simulink subsystem "WB"  (R2024b)
settings: Solver=VariableStepAuto  StartTime=0.0  StopTime=10.0  RelTol=1e-3
libraries: hdlsllib x1
settings Model: Creator=stefano  LastModifiedBy=stefano

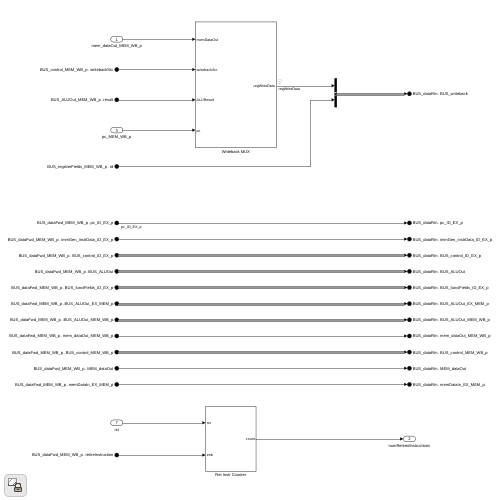
[thumbnail: Simulink's stored preview of the top-level diagram]
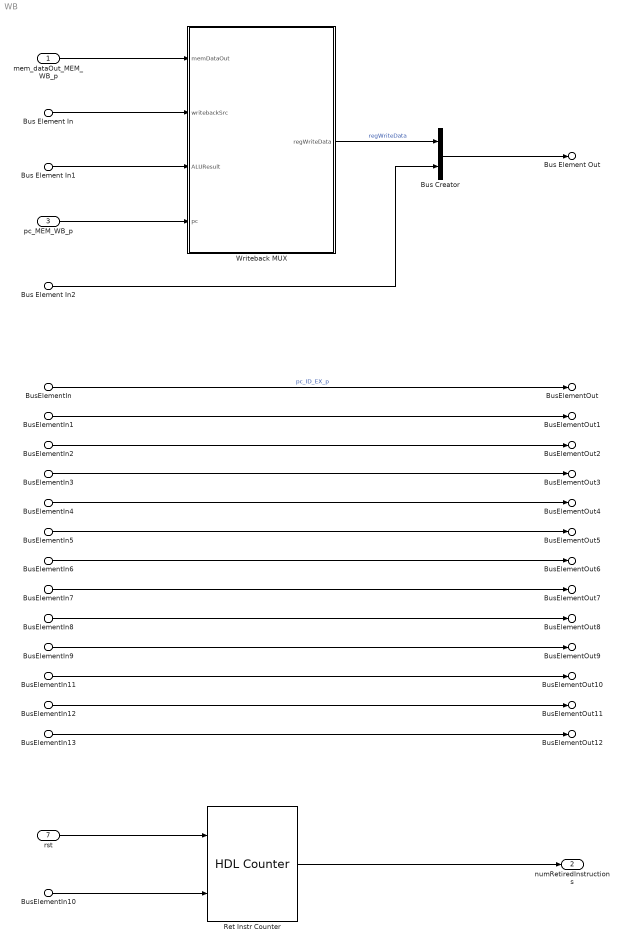
== system WB ==
  mem_dataOut_MEM_WB_p : Inport
  Bus Element In1 : Inport  Port=2  PortName=BUS_ALUOut_MEM_WB_p  Element=result
  pc_MEM_WB_p : Inport  Port=3
  Bus Element In : Inport  Port=4  PortName=BUS_control_MEM_WB_p  Element=writebackSrc
  Bus Element In2 : Inport  Port=5  PortName=BUS_registerFields_MEM_WB_p  Element=rd
  BusElementIn : Inport  Port=6  PortName=BUS_dataFwd_MEM_WB_p  Element=pc_ID_EX_p
  BusElementIn1 : Inport  Port=6  PortName=BUS_dataFwd_MEM_WB_p  Element=immGen_instrData_ID_EX_p
  BusElementIn2 : Inport  Port=6  PortName=BUS_dataFwd_MEM_WB_p  Element=BUS_control_ID_EX_p
  BusElementIn3 : Inport  Port=6  PortName=BUS_dataFwd_MEM_WB_p  Element=BUS_ALUOut
  BusElementIn4 : Inport  Port=6  PortName=BUS_dataFwd_MEM_WB_p  Element=BUS_functFields_ID_EX_p
  BusElementIn5 : Inport  Port=6  PortName=BUS_dataFwd_MEM_WB_p  Element=BUS_ALUOut_EX_MEM_p
  BusElementIn6 : Inport  Port=6  PortName=BUS_dataFwd_MEM_WB_p  Element=BUS_ALUOut_MEM_WB_p
  BusElementIn7 : Inport  Port=6  PortName=BUS_dataFwd_MEM_WB_p  Element=mem_dataOut_MEM_WB_p
  BusElementIn8 : Inport  Port=6  PortName=BUS_dataFwd_MEM_WB_p  Element=BUS_control_MEM_WB_p
  BusElementIn9 : Inport  Port=6  PortName=BUS_dataFwd_MEM_WB_p  Element=MEM_dataOut
  BusElementIn10 : Inport  Port=6  PortName=BUS_dataFwd_MEM_WB_p  Element=retireInstruction
  BusElementIn11 : Inport  Port=6  PortName=BUS_dataFwd_MEM_WB_p  Element=memDataIn_EX_MEM_p
  BusElementIn12 : Inport  Port=6  PortName=BUS_dataFwd_MEM_WB_p  Element=BUS_functFields_EX_MEM_p
  BusElementIn13 : Inport  Port=6  PortName=BUS_dataFwd_MEM_WB_p  Element=BUS_control_EX_MEM_p
  rst : Inport  Port=7
  Bus Creator : BusCreator  Inputs=2
  Ret Instr Counter : hdlsllib/Sources/HDL Counter  CountType=Count limited  CountInit=0  CountStep=1  CountMax=2^32-1  CountFromType=Initial value  CountFrom=0  CountResetPort=on  CountLoadPort=off  CountEnbPort=on  CountDirPort=off  CountHitOutputPort=off  CountDataType=Unsigned  CountWordLen=32  CountFracLen=0  CountSampTime=1
  Writeback MUX : Subsystem
  Bus Element Out : Outport  PortName=BUS_dataRtn  Element=BUS_writeback
  BusElementOut : Outport  PortName=BUS_dataRtn  Element=pc_ID_EX_p
  BusElementOut1 : Outport  PortName=BUS_dataRtn  Element=immGen_instrData_ID_EX_p
  BusElementOut2 : Outport  PortName=BUS_dataRtn  Element=BUS_control_ID_EX_p
  BusElementOut3 : Outport  PortName=BUS_dataRtn  Element=BUS_ALUOut
  BusElementOut4 : Outport  PortName=BUS_dataRtn  Element=BUS_functFields_ID_EX_p
  BusElementOut5 : Outport  PortName=BUS_dataRtn  Element=BUS_ALUOut_EX_MEM_p
  BusElementOut6 : Outport  PortName=BUS_dataRtn  Element=BUS_ALUOut_MEM_WB_p
  BusElementOut7 : Outport  PortName=BUS_dataRtn  Element=mem_dataOut_MEM_WB_p
  BusElementOut8 : Outport  PortName=BUS_dataRtn  Element=BUS_control_MEM_WB_p
  BusElementOut9 : Outport  PortName=BUS_dataRtn  Element=MEM_dataOut
  BusElementOut10 : Outport  PortName=BUS_dataRtn  Element=memDataIn_EX_MEM_p
  BusElementOut11 : Outport  PortName=BUS_dataRtn  Element=BUS_functFields_EX_MEM_p
  BusElementOut12 : Outport  PortName=BUS_dataRtn  Element=BUS_control_EX_MEM_p
  numRetiredInstructions : Outport  Port=2
  wires:
  Writeback MUX/1(regWriteData) -> Bus Creator/1  "regWriteData"
  Bus Element In2/1 -> Bus Creator/2
  pc_MEM_WB_p/1 -> Writeback MUX/4(pc)
  mem_dataOut_MEM_WB_p/1 -> Writeback MUX/1(memDataOut)
  Bus Element In1/1 -> Writeback MUX/3(ALUResult)
  Bus Element In/1 -> Writeback MUX/2(writebackSrc)
  Bus Creator/1 -> Bus Element Out/1
  BusElementIn/1 -> BusElementOut/1  "pc_ID_EX_p"
  BusElementIn1/1 -> BusElementOut1/1
  BusElementIn2/1 -> BusElementOut2/1
  BusElementIn3/1 -> BusElementOut3/1
  BusElementIn4/1 -> BusElementOut4/1
  BusElementIn5/1 -> BusElementOut5/1
  BusElementIn6/1 -> BusElementOut6/1
  BusElementIn7/1 -> BusElementOut7/1
  BusElementIn8/1 -> BusElementOut8/1
  BusElementIn9/1 -> BusElementOut9/1
  rst/1 -> Ret Instr Counter/1
  Ret Instr Counter/1 -> numRetiredInstructions/1
  BusElementIn10/1 -> Ret Instr Counter/2
  BusElementIn11/1 -> BusElementOut10/1
  BusElementIn12/1 -> BusElementOut11/1
  BusElementIn13/1 -> BusElementOut12/1

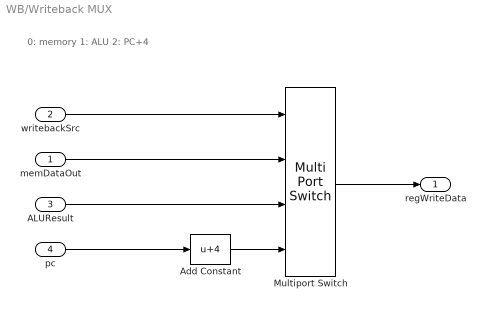
== system WB/Writeback MUX ==
  note: 0: memory
      | 1: ALU
      | 2: PC+4
  memDataOut : Inport
  writebackSrc : Inport  Port=2
  ALUResult : Inport  Port=3
  pc : Inport  Port=4
  Add Constant : Bias  Bias=4  SaturateOnIntegerOverflow=off
  Multiport Switch : MultiPortSwitch  DataPortOrder=Zero-based contiguous  zeroidx=on  SaturateOnIntegerOverflow=off  InputSameDT=off
  regWriteData : Outport
  wires:
  pc/1 -> Add Constant/1
  Add Constant/1 -> Multiport Switch/4
  writebackSrc/1 -> Multiport Switch/1
  ALUResult/1 -> Multiport Switch/3
  Multiport Switch/1 -> regWriteData/1
  memDataOut/1 -> Multiport Switch/2
